simulink model "msim"  (R2024b)
settings: Solver=VariableStepAuto  StartTime=tspan(1)  StopTime=tspan(2)  RelTol=1e-3
values from neighbouring files (symbols this model uses):
  den = [1 1 0.2]    [main.m]
  num = 0.1    [main.m]
  step_t = 5    [main.m]
  u_des = 1    [main.m]
settings Model: Creator=markminerov  LastModifiedBy=markminerov

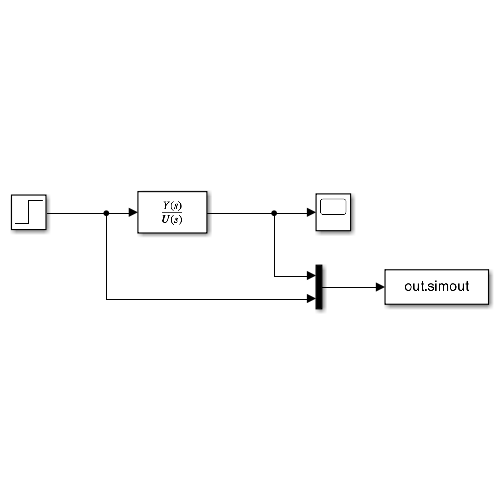
[thumbnail: Simulink's stored preview of the top-level diagram]
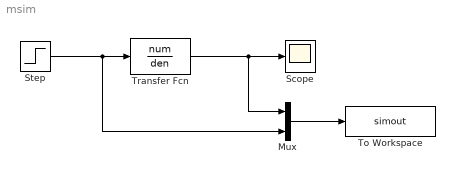
== system msim ==
  Mux : Mux  Inputs=2
  Scope : Scope
  Step : Step  Time=step_t  After=u_des  SampleTime=0
  To Workspace : ToWorkspace  VariableName=simout  SaveFormat=Timeseries  SampleTime=-1
  Transfer Fcn : TransferFcn  Numerator=num  Denominator=den
  wires:
  Step/1 -> Mux/2, Transfer Fcn/1
  Transfer Fcn/1 -> Mux/1, Scope/1
  Mux/1 -> To Workspace/1
